simulink model "CTRL_SPECCTRL_FF_BSTOP_test"  (R2024b)
settings: Solver=VariableStepAuto  StartTime=0.0  StopTime=10.0  RelTol=1e-3
libraries: CTRL_SPECCTRL_FF_BSTOP x1
settings Model: Creator=blatak  LastModifiedBy=blatak

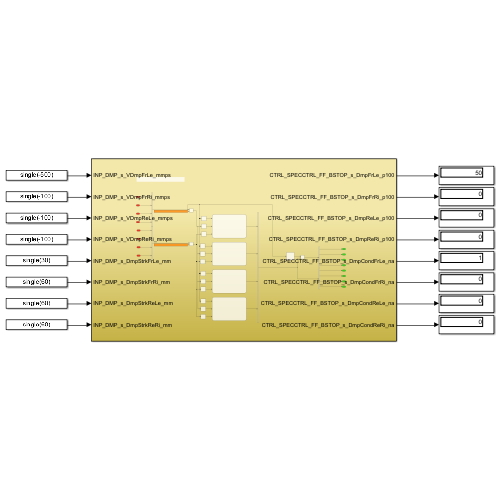
[thumbnail: Simulink's stored preview of the top-level diagram]
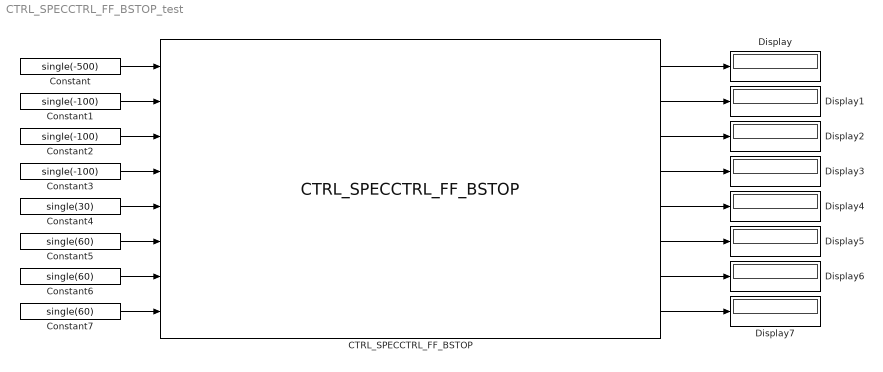
== system CTRL_SPECCTRL_FF_BSTOP_test ==
  CTRL_SPECCTRL_FF_BSTOP : CTRL_SPECCTRL_FF_BSTOP/CTRL_SPECCTRL_FF_BSTOP  SystemSampleTime=-1  VariantActivationTime=update diagram  AllowFlexibleInterface=on  Latency=0  AutoFrameSizeCalculation=off
      link override 1-D Lookup Table: BreakpointsForDimension1=CTRL_SPECCTRL_FF_BSTOP_px_vDmp_mmps  Table=CTRL_SPECCTRL_FF_BSTOP_py_Dmp_p100
  Constant : Constant  Value=single(-500)
  Constant1 : Constant  Value=single(-100)
  Constant2 : Constant  Value=single(-100)
  Constant3 : Constant  Value=single(-100)
  Constant4 : Constant  Value=single(30)
  Constant5 : Constant  Value=single(60)
  Constant6 : Constant  Value=single(60)
  Constant7 : Constant  Value=single(60)
  Display{,1..7} (8 alike) : Display
  wires:
  CTRL_SPECCTRL_FF_BSTOP/1 -> Display/1
  CTRL_SPECCTRL_FF_BSTOP/2 -> Display1/1
  CTRL_SPECCTRL_FF_BSTOP/3 -> Display2/1
  CTRL_SPECCTRL_FF_BSTOP/4 -> Display3/1
  Constant/1 -> CTRL_SPECCTRL_FF_BSTOP/1
  Constant1/1 -> CTRL_SPECCTRL_FF_BSTOP/2
  Constant2/1 -> CTRL_SPECCTRL_FF_BSTOP/3
  Constant3/1 -> CTRL_SPECCTRL_FF_BSTOP/4
  Constant4/1 -> CTRL_SPECCTRL_FF_BSTOP/5
  Constant5/1 -> CTRL_SPECCTRL_FF_BSTOP/6
  Constant6/1 -> CTRL_SPECCTRL_FF_BSTOP/7
  Constant7/1 -> CTRL_SPECCTRL_FF_BSTOP/8
  CTRL_SPECCTRL_FF_BSTOP/5 -> Display4/1
  CTRL_SPECCTRL_FF_BSTOP/6 -> Display5/1
  CTRL_SPECCTRL_FF_BSTOP/7 -> Display6/1
  CTRL_SPECCTRL_FF_BSTOP/8 -> Display7/1
